simulink model "lab9"  (R2023a)
settings: Solver=VariableStepAuto  StartTime=0.0  StopTime=20  RelTol=1e-3
libraries: simulink x1
settings Model: Creator=mluser  LastModifiedBy=laura

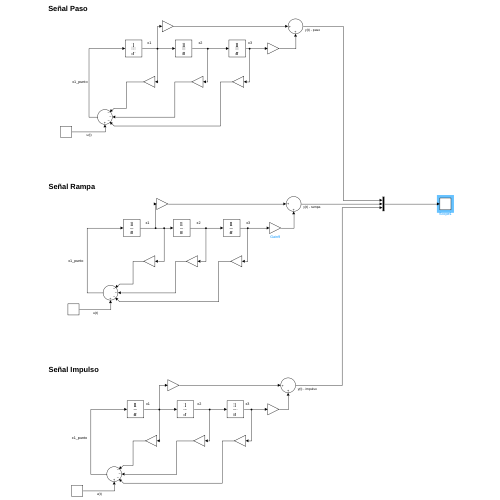
[thumbnail: Simulink's stored preview of the top-level diagram]
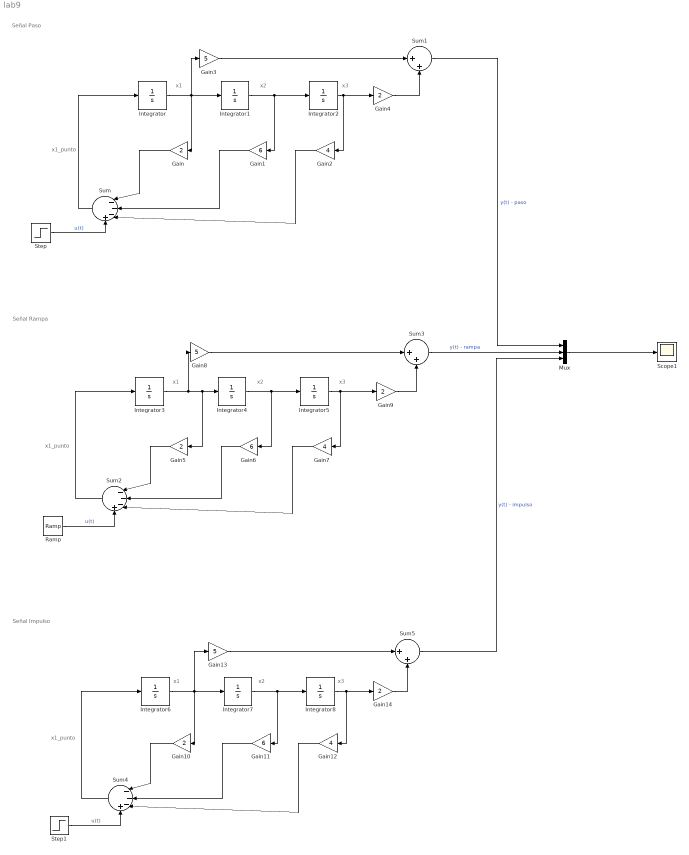
== system lab9 ==
  note: Señal Paso
  note: x1_punto
  note: x1
  note: x2
  note: x3
  note: x1
  note: x1_punto
  note: x3
  note: x2
  note: x1
  note: x1_punto
  note: x3
  note: x2
  note: Señal Rampa
  note: Señal Impulso
  Gain{,4..5,9..10,14} (6 alike) : Gain  Gain=2
  Gain1 : Gain  Gain=6
  Gain11 : Gain  Gain=6
  Gain12 : Gain  Gain=4
  Gain13 : Gain  Gain=5
  Gain2 : Gain  Gain=4
  Gain3 : Gain  Gain=5
  Gain6 : Gain  Gain=6
  Gain7 : Gain  Gain=4
  Gain8 : Gain  Gain=5
  Integrator{,1..8} (9 alike) : Integrator
  Mux : Mux  Inputs=3
  Ramp : simulink/Sources/Ramp  slope=1  start=0  InitialOutput=0
  Scope1 : Scope
  Step : Step  SampleTime=0
  Step1 : Step  Time=.2  Before=1  After=0  SampleTime=0
  Sum : Sum  Inputs=|---+
  Sum1 : Sum  Inputs=|++
  Sum2 : Sum  Inputs=|---+
  Sum3 : Sum  Inputs=|++
  Sum4 : Sum  Inputs=|---+
  Sum5 : Sum  Inputs=|++
  wires:
  Integrator/1 -> Gain/1, Gain3/1, Integrator1/1
  Integrator1/1 -> Gain1/1, Integrator2/1
  Sum/1 -> Integrator/1
  Gain/1 -> Sum/1
  Gain1/1 -> Sum/2
  Integrator2/1 -> Gain4/1, Gain2/1
  Gain2/1 -> Sum/3
  Gain3/1 -> Sum1/1
  Gain4/1 -> Sum1/2
  Step/1 -> Sum/4  "u(t)"
  Gain5/1 -> Sum2/1
  Gain8/1 -> Sum3/1
  Gain9/1 -> Sum3/2
  Integrator5/1 -> Gain9/1, Gain7/1
  Gain7/1 -> Sum2/3
  Ramp/1 -> Sum2/4  "u(t)"
  Integrator4/1 -> Gain6/1, Integrator5/1
  Sum2/1 -> Integrator3/1
  Gain6/1 -> Sum2/2
  Integrator3/1 -> Gain5/1, Integrator4/1, Gain8/1
  Gain10/1 -> Sum4/1
  Gain13/1 -> Sum5/1
  Gain14/1 -> Sum5/2
  Integrator8/1 -> Gain14/1, Gain12/1
  Gain12/1 -> Sum4/3
  Step1/1 -> Sum4/4  "u(t)"
  Integrator7/1 -> Gain11/1, Integrator8/1
  Sum4/1 -> Integrator6/1
  Gain11/1 -> Sum4/2
  Integrator6/1 -> Gain10/1, Gain13/1, Integrator7/1
  Sum3/1 -> Mux/2  "y(t) - rampa"
  Mux/1 -> Scope1/1
  Sum5/1 -> Mux/3  "y(t) - impulso"
  Sum1/1 -> Mux/1  "y(t) - paso"
